simulink model "simulation"  (R2019a)
settings: Solver=VariableStepAuto  StartTime=0.0  StopTime=1000  RelTol=1e-3
values from neighbouring files (symbols this model uses):
  To = 9.577    [data.m]
  Ts = 1    [data.m]
undefined symbols (not defined in the file or in its folder): DEN_Gbasic, NUM_Gbasic
libraries: simulink x1
settings Model: Creator=natal  LastModifiedBy=natal

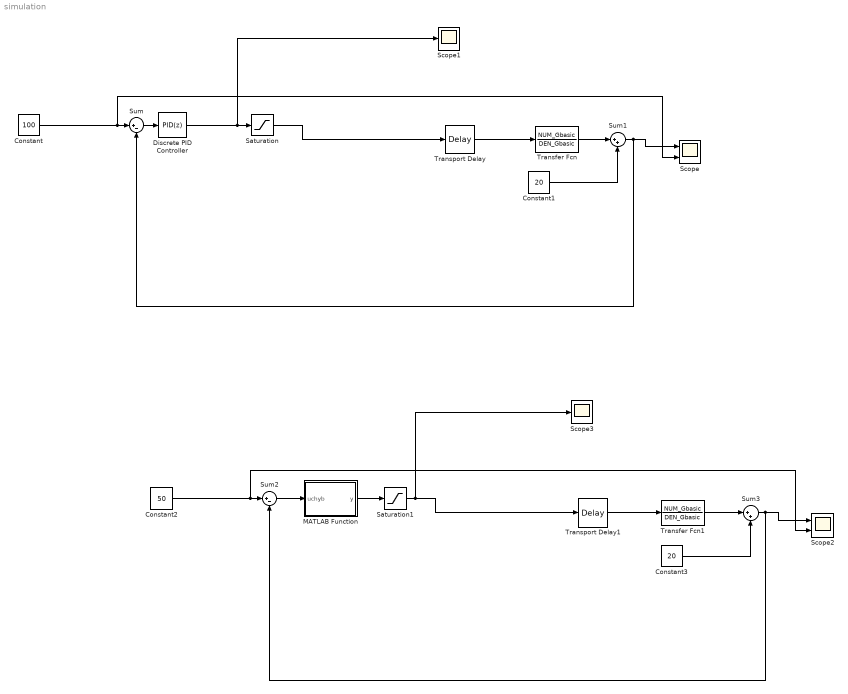
== system simulation ==
  Constant : Constant  Value=100
  Constant1 : Constant  Value=20
  Constant2 : Constant  Value=50
  Constant3 : Constant  Value=20
  Discrete PID Controller : simulink/Continuous/PID Controller  Controller=PID  Form=Parallel  TimeDomain=Discrete-time  SampleTime=Ts  IntegratorMethod=Trapezoidal  FilterMethod=Trapezoidal  ControllerParametersSource=internal  P=2.07  I=0.047  D=0  UseFilter=off  N=0.0371482559446449  TunerSelectOption=Transfer Function Based (PID Tuner App)  ZeroCross=off  InitialConditionSource=internal  InitialConditionForIntegrator=0  InitialConditionForFilter=0  DifferentiatorICPrevScaledInput=0  ExternalReset=none  TrackingMode=off  Kt=1  LimitOutput=on  UpperSaturationLimit=230  LowerSaturationLimit=0  LinearizeAsGain=off  AntiWindupMode=back-calculation  Kb=2  POutMin=[]  POutMax=[]  IOutMin=[]  IOutMax=[]  DOutMin=[]  DOutMax=[]  NOutMin=[]  NOutMax=[]  SumOutMin=[]  SumOutMax=[]  SaturationOutMin=[]  SaturationOutMax=[]  PParamMin=[]  PParamMax=[]  IParamMin=[]  IParamMax=[]  DParamMin=[]  DParamMax=[]  NParamMin=[]  NParamMax=[]  KbParamMin=[]  KbParamMax=[]  KtParamMin=[]  KtParamMax=[]  KbOutMin=[]  KbOutMax=[]  KtOutMin=[]  KtOutMax=[]  IntegratorOutMin=[]  IntegratorOutMax=[]  FilterOutMin=[]  FilterOutMax=[]  SumI1OutMin=[]  SumI1OutMax=[]  SumI2OutMin=[]  SumI2OutMax=[]  SumI3OutMin=[]  SumI3OutMax=[]  SumI4OutMin=[]  SumI4OutMax=[]  SumDOutMin=[]  SumDOutMax=[]  DifferentiatorOutMin=[]  DifferentiatorOutMax=[]  FilterDiffOutCoefMin=[]  FilterDiffOutCoefMax=[]  ReciprocalOutMin=[]  ReciprocalOutMax=[]  SumDenOutMin=[]  SumDenOutMax=[]  SumNumOutMin=[]  SumNumOutMax=[]  DivideOutMin=[]  DivideOutMax=[]  IntegratorContinuousStateAttributes=''  IntegratorStateMustResolveToSignalObject=off  IntegratorRTWStateStorageClass=Auto  FilterContinuousStateAttributes=''  FilterStateMustResolveToSignalObject=off  FilterRTWStateStorageClass=Auto  ParallelPVariant=InternalParameters  IdealPVariant=Disabled  IVariant=InternalParameters  DVariant=InternalParameters  IntegratorVariant=Discrete  SatVariant=Enabled  AWVariant=BackCalculation  PCopyVariant=Disabled  TRVariant=Disabled  FdbkBlocksVariant=Feedback  IdealPFdbkVariant=Passthrough  SatFdbkVariant=Enabled  DerivativeFilterVariant=Differentiator  NVariant=Passthrough  NCopyVariant=Disabled_SignalSpec  FilterICVariant=InternalICsDifferentiator  IntegratorICVariant=InternalICs  ExternalResetVariant=Disabled  TRSumVariant=Passthrough  SumFdbkVariant=Enabled  SumVariant=Sum_PID
  MATLAB Function : MATLAB Function  TreatAsAtomicUnit=on
  Saturation : Saturate  UpperLimit=230  LowerLimit=0
  Saturation1 : Saturate  UpperLimit=230  LowerLimit=0
  Scope : Scope  NumInputPorts=2
  Scope1 : Scope
  Scope2 : Scope  NumInputPorts=2
  Scope3 : Scope
  Sum : Sum  Inputs=|+-
  Sum1 : Sum  Inputs=|++
  Sum2 : Sum  Inputs=|+-
  Sum3 : Sum  Inputs=|++
  Transfer Fcn : TransferFcn  Numerator=NUM_Gbasic  Denominator=DEN_Gbasic
  Transfer Fcn1 : TransferFcn  Numerator=NUM_Gbasic  Denominator=DEN_Gbasic
  Transport Delay : TransportDelay  DelayTime=To
  Transport Delay1 : TransportDelay  DelayTime=To
  wires:
  Sum/1 -> Discrete PID Controller/1
  Constant/1 -> Scope/2, Sum/1
  Constant1/1 -> Sum1/2
  Sum1/1 -> Sum/2, Scope/1
  Saturation/1 -> Transport Delay/1
  Transfer Fcn/1 -> Sum1/1
  Transport Delay/1 -> Transfer Fcn/1
  Discrete PID Controller/1 -> Scope1/1, Saturation/1
  Constant2/1 -> Scope2/2, Sum2/1
  Saturation1/1 -> Scope3/1, Transport Delay1/1
  Sum3/1 -> Sum2/2, Scope2/1
  Constant3/1 -> Sum3/2
  MATLAB Function/1(y) -> Saturation1/1
  Sum2/1 -> MATLAB Function/1(uchyb)
  Transport Delay1/1 -> Transfer Fcn1/1
  Transfer Fcn1/1 -> Sum3/1

== matlab function simulation/MATLAB Function ==
  settings: updateMethod=DISCRETE
  data: uchyb input; y output
function y = fcn(uchyb)
% Deklaracja ststycznych wartości
persistent pop_uchyb;
if isempty(pop_uchyb)
    pop_uchyb = 0;
end

persistent pop_calka;
if isempty(pop_calka)
    pop_calka = 0;
end
persistent pop_u;
if isempty(pop_u)
    pop_u = 0;
end

dt = 1;
Kp = 2.07;
Ki = 0.047;
Kd = 0;
%N = 0.056;
% Część proporcjonalna:
P = Kp*uchyb;

% Część całkująca:
if pop_u==230
    Ki=0;
end
calka = pop_calka + (uchyb+pop_uchyb) ;
pop_calka = calka;
I = Ki*calka*(dt/2);

% Człon rózniczkujący:
rozniczka = (uchyb - pop_uchyb)/dt; 
pop_uchyb=uchyb;
D = Kd*rozniczka;


% Suma wszystkich części:
u = P  + I + D;
pop_u=u;
y = u;
